simulink model "Copy_of_VTOLTiltrotor"  (R2024a)
settings: configuration reference "VTOLConfiguration" (kept outside this file)
undefined symbols (not defined in the file): airspeed, Battery, BCE12, BCE_Set_init, BMS_Controller_State, C, Cell10_P, Cell11_P, Cell12_P, Cell1_N, Cell1_P, Cell2_P, Cell3_P, Cell4_P, Cell5_P, Cell6_P, Cell7_P, Cell8_P, Cell9_P, Cell_Temperatures, Cell_Voltages, Charging_State, CityMission, control, controlParams, ControlSampleTime, CriticalTiltAngle, currentFactor, CV_Gain, ddx, ddy, ddz, Device_01, DiscIntNeverNeededParam, dx, dy, dz, Earth, env, F, F28379D_ADC_MaxCount, F28379D_ADC_Vmax, FixedWingMission, flightState, Foc_Ki_IxTcpu, Foc_Ki_S, Foc_Kp_I, Foc_Kp_S, fractalcoef, FSState, FWControlParams, HoverMission, I_cc, Ia_offset, Ib_offset, iniRoll, initPitch, iniYaw, IO334, IO334_DAC_Vmax ... (+55)
libraries: slrealtimeethercatlib x109, simulink x81, fl_lib x65, slpidlib x49, mcbcontrolslib x48, nesl_utility x43, speedgoatlib_hdlCoder_IO3xx x31, canmsglib x17, slrealtimeutilitieslib x13, mcbhdlplantlib x13, speedgoatlib_IO611 x12, dspstat3 x12
(part 18 of 20)

== system Copy_of_VTOLTiltrotor/Motor Control/Controller1/Controller_MIL/F28379D Firmware/Controller Algorithm/FOC/Speed Control MLD/PI_Controller_Speed ==
  Enable : Inport
  N_ref : Inport  Port=2
  N_fb : Inport  Port=3
  Kp_S : Inport  Port=4
  Ki_S : Inport  Port=5
  Discrete PI Controller with anti-windup & reset : slpidlib/PID Controller  Controller=PI  Form=Parallel  TimeDomain=Discrete-time  UseExternalTs=off  SampleTime=-1  IntegratorMethod=Forward Euler  FilterMethod=Forward Euler  ControllerParametersSource=external  P=1  I=1  UseKiTs=on  D=0  UseExternalDerivativeSource=off  N=100  UseFilter=on  TunerSelectOption=Transfer Function Based (PID Tuner App)  InitialConditionSource=external  InitialConditionForIntegrator=0  InitialConditionForFilter=0  DifferentiatorICPrevScaledInput=0  ExternalReset=level  TrackingMode=off  Kt=1  LimitOutput=on  SatLimitsSource=internal  UpperSaturationLimit=1  LowerSaturationLimit=-1  LinearizeAsGain=on  AntiWindupMode=clamping  Kb=1  LimitIntegrator=off  UpperIntegratorSaturationLimit=inf  LowerIntegratorSaturationLimit=-inf  RndMeth=Simplest  POutMin=[]  POutMax=[]  IOutMin=[]  IOutMax=[]  DOutMin=[]  DOutMax=[]  NOutMin=[]  NOutMax=[]  SumOutMin=[]  SumOutMax=[]  SaturationOutDataTypeStr=Inherit: Inherit via back propagation  SaturationOutMin=[]  SaturationOutMax=[]  PParamMin=[]  PParamMax=[]  IParamMin=[]  IParamMax=[]  DParamMin=[]  DParamMax=[]  NParamMin=[]  NParamMax=[]  KbParamMin=[]  KbParamMax=[]  KtParamMin=[]  KtParamMax=[]  KbOutMin=[]  KbOutMax=[]  KtOutMin=[]  KtOutMax=[]  IntegratorOutMin=[]  IntegratorOutMax=[]  FilterOutMin=[]  FilterOutMax=[]  SumI1OutMin=[]  SumI1OutMax=[]  SumI2OutMin=[]  SumI2OutMax=[]  SumI3OutMin=[]  SumI3OutMax=[]  SumI4OutMin=[]  SumI4OutMax=[]  SumDOutMin=[]  SumDOutMax=[]  DifferentiatorOutMin=[]  DifferentiatorOutMax=[]  FilterDiffOutCoefMin=[]  FilterDiffOutCoefMax=[]  ReciprocalOutMin=[]  ReciprocalOutMax=[]  SumDenOutMin=[]  SumDenOutMax=[]  SumNumOutMin=[]  SumNumOutMax=[]  DivideOutMin=[]  DivideOutMax=[]  UdiffTsProdOutMin=[]  UdiffTsProdOutMax=[]  NTsProdOutMin=[]  NTsProdOutMax=[]  UintegralTsProdOutMin=[]  UintegralTsProdOutMax=[]  UngainTsProdOutMin=[]  UngainTsProdOutMax=[]  ClampingZeroOutDataTypeStr=Inherit: Inherit via back propagation  ClampingZeroOutMin=[]  ClampingZeroOutMax=[]  FilterDenConstantOutDataTypeStr=Inherit: Inherit via back propagation  FilterDenConstantOutMin=[]  FilterDenConstantOutMax=[]  PCopyOutDataTypeStr=Inherit: Inherit via back propagation  PCopyOutMin=[]  PCopyOutMax=[]  NCopyOutDataTypeStr=Inherit: Inherit via back propagation  NCopyOutMin=[]  NCopyOutMax=[]  IntegratorContinuousStateAttributes=''  IntegratorStateMustResolveToSignalObject=off  IntegratorRTWStateStorageClass=Auto  FilterContinuousStateAttributes=''  FilterStateMustResolveToSignalObject=off  FilterRTWStateStorageClass=Auto  ParallelPVariant=ExternalParameters  IdealPVariant=Disabled  IVariant=ExternalParameters  DVariant=Disabled  IntegratorVariant=Discrete  SatVariant=Enabled  AWVariant=DiscClampingParallel  PCopyVariant=Disabled  TRVariant=Disabled  FdbkBlocksVariant=Forward  IdealPFdbkVariant=Disabled  SatFdbkVariant=Disabled  DerivativeFilterVariant=Disabled  NVariant=Disabled  NCopyVariant=Disabled_SignalSpec  FilterICVariant=Disabled  IntegratorICVariant=ExternalICs  ExternalResetVariant=ExternalReset  TRSumVariant=Passthrough  SumFdbkVariant=Disabled  SumVariant=Sum_PI  TsampFilterVariant=InternalTs  TsampNgainVariant=Passthrough  TsampIntegralVariant=Disabled_SignalSpec  ExternalSaturationOutDataTypeStr=Inherit: Same as second input  DerivativeSourceVariant=Disabled
  Ki2 : Constant  Value=0  OutDataTypeStr=single  SampleTime=-1
  Logical Operator : Logic  Operator=NOT  IconShape=distinctive  AllPortsSameDT=off  OutDataTypeStr=boolean
  Sum : Sum  Inputs=|+-  OutDataTypeStr=Inherit: Same as first input
  Iq_ref : Outport  VectorParamsAs1DForOutWhenUnconnected=off
  wires:
  Ki_S/1 -> Discrete PI Controller with anti-windup & reset/3
  Kp_S/1 -> Discrete PI Controller with anti-windup & reset/2
  Enable/1 -> Logical Operator/1
  Ki2/1 -> Discrete PI Controller with anti-windup & reset/5
  Logical Operator/1 -> Discrete PI Controller with anti-windup & reset/4
  Sum/1 -> Discrete PI Controller with anti-windup & reset/1
  N_ref/1 -> Sum/1
  N_fb/1 -> Sum/2
  Discrete PI Controller with anti-windup & reset/1 -> Iq_ref/1

== system Copy_of_VTOLTiltrotor/Motor Control/Controller1/Controller_MIL/F28379D Firmware/Controller Algorithm/FOC/Speed Control MLD/Speed_Ref_Selector ==
  Enable : Inport
  SpeedCommand : Inport  Port=2
  Speed_Ref_Open : Inport  Port=3
  IIR Filter : mcbcontrolslib/IIR Filter  VariantControl=Low Pass Filter  VariantSelect=Low-pass  FilterConstantInputType=Specify via dialog  Filter_constant=0.01  advancedSettings=off  Ts=50e-6  cutOff_freq=32.1525
  Switch : Switch  Criteria=u2 > Threshold  Threshold=0.5  SaturateOnIntegerOverflow=off  InputSameDT=off
  Speed_Ref_PU : Outport
  wires:
  SpeedCommand/1 -> Switch/1  "SpeedRef"
  Enable/1 -> Switch/2
  Speed_Ref_Open/1 -> Switch/3
  Switch/1 -> IIR Filter/1
  IIR Filter/1 -> Speed_Ref_PU/1

== system Copy_of_VTOLTiltrotor/Motor Control/Controller2/Controller_MIL/F28379D Firmware/Controller Algorithm/FOC/Current Control/Control_System ==
  Iab_meas_PU : Inport
  Pos_PU : Inport  Port=2
  Enable : Inport  Port=3
  Idq_ref_PU : Inport  Port=4
  SpeedRef : Inport  Port=5
  Kp_i : Inport  Port=6
  Ki_ixTcpu : Inport  Port=7
  Closed Loop Control : Subsystem
  Demux : Demux  Outputs=2
  NOT : Logic  Operator=NOT  IconShape=distinctive  AllPortsSameDT=off  OutDataTypeStr=boolean
  Open Loop Start-Up : Subsystem
  Output Scaling : Subsystem
  Switch : Switch  Criteria=u2 > Threshold  Threshold=0.5  SaturateOnIntegerOverflow=off  InputSameDT=off
  ModWave : Outport
  PWM_Enable : Outport  Port=2
  Idq_debug : Outport  Port=3  VectorParamsAs1DForOutWhenUnconnected=off
  wires:
  Open Loop Start-Up/1(PWM_Duty) -> Switch/3
  Switch/1 -> Output Scaling/1(PWM_Duty)
  Enable/1 -> Demux/1
  Demux/1 -> Closed Loop Control/Enable, Switch/2, NOT/1
  Demux/2 -> [EnablePWM], Open Loop Start-Up/1(<EnablePWM>)
  Iab_meas_PU/1 -> Closed Loop Control/1(Iab_meas_PU)
  Pos_PU/1 -> Closed Loop Control/2(Pos_PU)
  Idq_ref_PU/1 -> Closed Loop Control/3(Idq_ref_PU)  "idqref"
  [EnablePWM] -> Closed Loop Control/4(EnablePWM)
  Closed Loop Control/1(Idq_debug) -> Idq_debug/1
  Closed Loop Control/2(Vabc in PU) -> Switch/1
  Output Scaling/1(ModWave) -> ModWave/1
  Output Scaling/2(PWM_Enable) -> PWM_Enable/1
  [EnablePWM] -> Output Scaling/2(Enable)
  SpeedRef/1 -> Open Loop Start-Up/2(SpeedRef)
  NOT/1 -> Open Loop Start-Up/Enable
  Ki_ixTcpu/1 -> Closed Loop Control/6(Ki_ixTcpu)
  Kp_i/1 -> Closed Loop Control/5(Kp_i)

== system Copy_of_VTOLTiltrotor/Motor Control/Controller2/Controller_MIL/F28379D Firmware/Controller Algorithm/FOC/Speed Control MLD/PI_Controller_Speed ==
  Enable : Inport
  N_ref : Inport  Port=2
  N_fb : Inport  Port=3
  Kp_S : Inport  Port=4
  Ki_S : Inport  Port=5
  Discrete PI Controller with anti-windup & reset : slpidlib/PID Controller  Controller=PI  Form=Parallel  TimeDomain=Discrete-time  UseExternalTs=off  SampleTime=-1  IntegratorMethod=Forward Euler  FilterMethod=Forward Euler  ControllerParametersSource=external  P=1  I=1  UseKiTs=on  D=0  UseExternalDerivativeSource=off  N=100  UseFilter=on  TunerSelectOption=Transfer Function Based (PID Tuner App)  InitialConditionSource=external  InitialConditionForIntegrator=0  InitialConditionForFilter=0  DifferentiatorICPrevScaledInput=0  ExternalReset=level  TrackingMode=off  Kt=1  LimitOutput=on  SatLimitsSource=internal  UpperSaturationLimit=1  LowerSaturationLimit=-1  LinearizeAsGain=on  AntiWindupMode=clamping  Kb=1  LimitIntegrator=off  UpperIntegratorSaturationLimit=inf  LowerIntegratorSaturationLimit=-inf  RndMeth=Simplest  POutMin=[]  POutMax=[]  IOutMin=[]  IOutMax=[]  DOutMin=[]  DOutMax=[]  NOutMin=[]  NOutMax=[]  SumOutMin=[]  SumOutMax=[]  SaturationOutDataTypeStr=Inherit: Inherit via back propagation  SaturationOutMin=[]  SaturationOutMax=[]  PParamMin=[]  PParamMax=[]  IParamMin=[]  IParamMax=[]  DParamMin=[]  DParamMax=[]  NParamMin=[]  NParamMax=[]  KbParamMin=[]  KbParamMax=[]  KtParamMin=[]  KtParamMax=[]  KbOutMin=[]  KbOutMax=[]  KtOutMin=[]  KtOutMax=[]  IntegratorOutMin=[]  IntegratorOutMax=[]  FilterOutMin=[]  FilterOutMax=[]  SumI1OutMin=[]  SumI1OutMax=[]  SumI2OutMin=[]  SumI2OutMax=[]  SumI3OutMin=[]  SumI3OutMax=[]  SumI4OutMin=[]  SumI4OutMax=[]  SumDOutMin=[]  SumDOutMax=[]  DifferentiatorOutMin=[]  DifferentiatorOutMax=[]  FilterDiffOutCoefMin=[]  FilterDiffOutCoefMax=[]  ReciprocalOutMin=[]  ReciprocalOutMax=[]  SumDenOutMin=[]  SumDenOutMax=[]  SumNumOutMin=[]  SumNumOutMax=[]  DivideOutMin=[]  DivideOutMax=[]  UdiffTsProdOutMin=[]  UdiffTsProdOutMax=[]  NTsProdOutMin=[]  NTsProdOutMax=[]  UintegralTsProdOutMin=[]  UintegralTsProdOutMax=[]  UngainTsProdOutMin=[]  UngainTsProdOutMax=[]  ClampingZeroOutDataTypeStr=Inherit: Inherit via back propagation  ClampingZeroOutMin=[]  ClampingZeroOutMax=[]  FilterDenConstantOutDataTypeStr=Inherit: Inherit via back propagation  FilterDenConstantOutMin=[]  FilterDenConstantOutMax=[]  PCopyOutDataTypeStr=Inherit: Inherit via back propagation  PCopyOutMin=[]  PCopyOutMax=[]  NCopyOutDataTypeStr=Inherit: Inherit via back propagation  NCopyOutMin=[]  NCopyOutMax=[]  IntegratorContinuousStateAttributes=''  IntegratorStateMustResolveToSignalObject=off  IntegratorRTWStateStorageClass=Auto  FilterContinuousStateAttributes=''  FilterStateMustResolveToSignalObject=off  FilterRTWStateStorageClass=Auto  ParallelPVariant=ExternalParameters  IdealPVariant=Disabled  IVariant=ExternalParameters  DVariant=Disabled  IntegratorVariant=Discrete  SatVariant=Enabled  AWVariant=DiscClampingParallel  PCopyVariant=Disabled  TRVariant=Disabled  FdbkBlocksVariant=Forward  IdealPFdbkVariant=Disabled  SatFdbkVariant=Disabled  DerivativeFilterVariant=Disabled  NVariant=Disabled  NCopyVariant=Disabled_SignalSpec  FilterICVariant=Disabled  IntegratorICVariant=ExternalICs  ExternalResetVariant=ExternalReset  TRSumVariant=Passthrough  SumFdbkVariant=Disabled  SumVariant=Sum_PI  TsampFilterVariant=InternalTs  TsampNgainVariant=Passthrough  TsampIntegralVariant=Disabled_SignalSpec  ExternalSaturationOutDataTypeStr=Inherit: Same as second input  DerivativeSourceVariant=Disabled
  Ki2 : Constant  Value=0  OutDataTypeStr=single  SampleTime=-1
  Logical Operator : Logic  Operator=NOT  IconShape=distinctive  AllPortsSameDT=off  OutDataTypeStr=boolean
  Sum : Sum  Inputs=|+-  OutDataTypeStr=Inherit: Same as first input
  Iq_ref : Outport  VectorParamsAs1DForOutWhenUnconnected=off
  wires:
  Ki_S/1 -> Discrete PI Controller with anti-windup & reset/3
  Kp_S/1 -> Discrete PI Controller with anti-windup & reset/2
  Enable/1 -> Logical Operator/1
  Ki2/1 -> Discrete PI Controller with anti-windup & reset/5
  Logical Operator/1 -> Discrete PI Controller with anti-windup & reset/4
  Sum/1 -> Discrete PI Controller with anti-windup & reset/1
  N_ref/1 -> Sum/1
  N_fb/1 -> Sum/2
  Discrete PI Controller with anti-windup & reset/1 -> Iq_ref/1

== system Copy_of_VTOLTiltrotor/Motor Control/Controller2/Controller_MIL/F28379D Firmware/Controller Algorithm/FOC/Speed Control MLD/Speed_Ref_Selector ==
  Enable : Inport
  SpeedCommand : Inport  Port=2
  Speed_Ref_Open : Inport  Port=3
  IIR Filter : mcbcontrolslib/IIR Filter  VariantControl=Low Pass Filter  VariantSelect=Low-pass  FilterConstantInputType=Specify via dialog  Filter_constant=0.01  advancedSettings=off  Ts=50e-6  cutOff_freq=32.1525
  Switch : Switch  Criteria=u2 > Threshold  Threshold=0.5  SaturateOnIntegerOverflow=off  InputSameDT=off
  Speed_Ref_PU : Outport
  wires:
  SpeedCommand/1 -> Switch/1  "SpeedRef"
  Enable/1 -> Switch/2
  Speed_Ref_Open/1 -> Switch/3
  Switch/1 -> IIR Filter/1
  IIR Filter/1 -> Speed_Ref_PU/1

== system Copy_of_VTOLTiltrotor/Motor Control/Controller3/Controller_MIL/F28379D Firmware/Controller Algorithm/FOC/Current Control/Control_System ==
  Iab_meas_PU : Inport
  Pos_PU : Inport  Port=2
  Enable : Inport  Port=3
  Idq_ref_PU : Inport  Port=4
  SpeedRef : Inport  Port=5
  Kp_i : Inport  Port=6
  Ki_ixTcpu : Inport  Port=7
  Closed Loop Control : Subsystem
  Demux : Demux  Outputs=2
  NOT : Logic  Operator=NOT  IconShape=distinctive  AllPortsSameDT=off  OutDataTypeStr=boolean
  Open Loop Start-Up : Subsystem
  Output Scaling : Subsystem
  Switch : Switch  Criteria=u2 > Threshold  Threshold=0.5  SaturateOnIntegerOverflow=off  InputSameDT=off
  ModWave : Outport
  PWM_Enable : Outport  Port=2
  Idq_debug : Outport  Port=3  VectorParamsAs1DForOutWhenUnconnected=off
  wires:
  Open Loop Start-Up/1(PWM_Duty) -> Switch/3
  Switch/1 -> Output Scaling/1(PWM_Duty)
  Enable/1 -> Demux/1
  Demux/1 -> Closed Loop Control/Enable, Switch/2, NOT/1
  Demux/2 -> [EnablePWM], Open Loop Start-Up/1(<EnablePWM>)
  Iab_meas_PU/1 -> Closed Loop Control/1(Iab_meas_PU)
  Pos_PU/1 -> Closed Loop Control/2(Pos_PU)
  Idq_ref_PU/1 -> Closed Loop Control/3(Idq_ref_PU)  "idqref"
  [EnablePWM] -> Closed Loop Control/4(EnablePWM)
  Closed Loop Control/1(Idq_debug) -> Idq_debug/1
  Closed Loop Control/2(Vabc in PU) -> Switch/1
  Output Scaling/1(ModWave) -> ModWave/1
  Output Scaling/2(PWM_Enable) -> PWM_Enable/1
  [EnablePWM] -> Output Scaling/2(Enable)
  SpeedRef/1 -> Open Loop Start-Up/2(SpeedRef)
  NOT/1 -> Open Loop Start-Up/Enable
  Ki_ixTcpu/1 -> Closed Loop Control/6(Ki_ixTcpu)
  Kp_i/1 -> Closed Loop Control/5(Kp_i)

== system Copy_of_VTOLTiltrotor/Motor Control/Controller3/Controller_MIL/F28379D Firmware/Controller Algorithm/FOC/Speed Control MLD/PI_Controller_Speed ==
  Enable : Inport
  N_ref : Inport  Port=2
  N_fb : Inport  Port=3
  Kp_S : Inport  Port=4
  Ki_S : Inport  Port=5
  Discrete PI Controller with anti-windup & reset : slpidlib/PID Controller  Controller=PI  Form=Parallel  TimeDomain=Discrete-time  UseExternalTs=off  SampleTime=-1  IntegratorMethod=Forward Euler  FilterMethod=Forward Euler  ControllerParametersSource=external  P=1  I=1  UseKiTs=on  D=0  UseExternalDerivativeSource=off  N=100  UseFilter=on  TunerSelectOption=Transfer Function Based (PID Tuner App)  InitialConditionSource=external  InitialConditionForIntegrator=0  InitialConditionForFilter=0  DifferentiatorICPrevScaledInput=0  ExternalReset=level  TrackingMode=off  Kt=1  LimitOutput=on  SatLimitsSource=internal  UpperSaturationLimit=1  LowerSaturationLimit=-1  LinearizeAsGain=on  AntiWindupMode=clamping  Kb=1  LimitIntegrator=off  UpperIntegratorSaturationLimit=inf  LowerIntegratorSaturationLimit=-inf  RndMeth=Simplest  POutMin=[]  POutMax=[]  IOutMin=[]  IOutMax=[]  DOutMin=[]  DOutMax=[]  NOutMin=[]  NOutMax=[]  SumOutMin=[]  SumOutMax=[]  SaturationOutDataTypeStr=Inherit: Inherit via back propagation  SaturationOutMin=[]  SaturationOutMax=[]  PParamMin=[]  PParamMax=[]  IParamMin=[]  IParamMax=[]  DParamMin=[]  DParamMax=[]  NParamMin=[]  NParamMax=[]  KbParamMin=[]  KbParamMax=[]  KtParamMin=[]  KtParamMax=[]  KbOutMin=[]  KbOutMax=[]  KtOutMin=[]  KtOutMax=[]  IntegratorOutMin=[]  IntegratorOutMax=[]  FilterOutMin=[]  FilterOutMax=[]  SumI1OutMin=[]  SumI1OutMax=[]  SumI2OutMin=[]  SumI2OutMax=[]  SumI3OutMin=[]  SumI3OutMax=[]  SumI4OutMin=[]  SumI4OutMax=[]  SumDOutMin=[]  SumDOutMax=[]  DifferentiatorOutMin=[]  DifferentiatorOutMax=[]  FilterDiffOutCoefMin=[]  FilterDiffOutCoefMax=[]  ReciprocalOutMin=[]  ReciprocalOutMax=[]  SumDenOutMin=[]  SumDenOutMax=[]  SumNumOutMin=[]  SumNumOutMax=[]  DivideOutMin=[]  DivideOutMax=[]  UdiffTsProdOutMin=[]  UdiffTsProdOutMax=[]  NTsProdOutMin=[]  NTsProdOutMax=[]  UintegralTsProdOutMin=[]  UintegralTsProdOutMax=[]  UngainTsProdOutMin=[]  UngainTsProdOutMax=[]  ClampingZeroOutDataTypeStr=Inherit: Inherit via back propagation  ClampingZeroOutMin=[]  ClampingZeroOutMax=[]  FilterDenConstantOutDataTypeStr=Inherit: Inherit via back propagation  FilterDenConstantOutMin=[]  FilterDenConstantOutMax=[]  PCopyOutDataTypeStr=Inherit: Inherit via back propagation  PCopyOutMin=[]  PCopyOutMax=[]  NCopyOutDataTypeStr=Inherit: Inherit via back propagation  NCopyOutMin=[]  NCopyOutMax=[]  IntegratorContinuousStateAttributes=''  IntegratorStateMustResolveToSignalObject=off  IntegratorRTWStateStorageClass=Auto  FilterContinuousStateAttributes=''  FilterStateMustResolveToSignalObject=off  FilterRTWStateStorageClass=Auto  ParallelPVariant=ExternalParameters  IdealPVariant=Disabled  IVariant=ExternalParameters  DVariant=Disabled  IntegratorVariant=Discrete  SatVariant=Enabled  AWVariant=DiscClampingParallel  PCopyVariant=Disabled  TRVariant=Disabled  FdbkBlocksVariant=Forward  IdealPFdbkVariant=Disabled  SatFdbkVariant=Disabled  DerivativeFilterVariant=Disabled  NVariant=Disabled  NCopyVariant=Disabled_SignalSpec  FilterICVariant=Disabled  IntegratorICVariant=ExternalICs  ExternalResetVariant=ExternalReset  TRSumVariant=Passthrough  SumFdbkVariant=Disabled  SumVariant=Sum_PI  TsampFilterVariant=InternalTs  TsampNgainVariant=Passthrough  TsampIntegralVariant=Disabled_SignalSpec  ExternalSaturationOutDataTypeStr=Inherit: Same as second input  DerivativeSourceVariant=Disabled
  Ki2 : Constant  Value=0  OutDataTypeStr=single  SampleTime=-1
  Logical Operator : Logic  Operator=NOT  IconShape=distinctive  AllPortsSameDT=off  OutDataTypeStr=boolean
  Sum : Sum  Inputs=|+-  OutDataTypeStr=Inherit: Same as first input
  Iq_ref : Outport  VectorParamsAs1DForOutWhenUnconnected=off
  wires:
  Ki_S/1 -> Discrete PI Controller with anti-windup & reset/3
  Kp_S/1 -> Discrete PI Controller with anti-windup & reset/2
  Enable/1 -> Logical Operator/1
  Ki2/1 -> Discrete PI Controller with anti-windup & reset/5
  Logical Operator/1 -> Discrete PI Controller with anti-windup & reset/4
  Sum/1 -> Discrete PI Controller with anti-windup & reset/1
  N_ref/1 -> Sum/1
  N_fb/1 -> Sum/2
  Discrete PI Controller with anti-windup & reset/1 -> Iq_ref/1

== system Copy_of_VTOLTiltrotor/Motor Control/Controller3/Controller_MIL/F28379D Firmware/Controller Algorithm/FOC/Speed Control MLD/Speed_Ref_Selector ==
  Enable : Inport
  SpeedCommand : Inport  Port=2
  Speed_Ref_Open : Inport  Port=3
  IIR Filter : mcbcontrolslib/IIR Filter  VariantControl=Low Pass Filter  VariantSelect=Low-pass  FilterConstantInputType=Specify via dialog  Filter_constant=0.01  advancedSettings=off  Ts=50e-6  cutOff_freq=32.1525
  Switch : Switch  Criteria=u2 > Threshold  Threshold=0.5  SaturateOnIntegerOverflow=off  InputSameDT=off
  Speed_Ref_PU : Outport
  wires:
  SpeedCommand/1 -> Switch/1  "SpeedRef"
  Enable/1 -> Switch/2
  Speed_Ref_Open/1 -> Switch/3
  Switch/1 -> IIR Filter/1
  IIR Filter/1 -> Speed_Ref_PU/1

== system Copy_of_VTOLTiltrotor/Battery Management System/Battery/HW Interface/BCE - HIL/Battery Cell Emulator/BCE Write /Subsystem/BCE Write /Enable until confirmed ==
  global enable : Inport
  D1 : Inport  Port=2
  D2 : Inport  Port=3
  D3 : Inport  Port=4
  D4 : Inport  Port=5
  D5 : Inport  Port=6
  D6 : Inport  Port=7
  D7 : Inport  Port=8
  D8 : Inport  Port=9
  D9 : Inport  Port=10
  D10 : Inport  Port=11
  D11 : Inport  Port=12
  D12 : Inport  Port=13
  Compare To Constant{,1..11} (12 alike) : simulink/Logic and Bit Operations/Compare To Constant  relop===  const=2  OutDataTypeStr=boolean
  Data Type Conversion : DataTypeConversion  OutDataTypeStr=int32  SaturateOnIntegerOverflow=off  RndMeth=Floor
  Logical Operator : Logic  Operator=NAND  Inputs=12  AllPortsSameDT=off  OutDataTypeStr=boolean
  Logical Operator1 : Logic  AllPortsSameDT=off  OutDataTypeStr=boolean
  Logical Operator2 : Logic  Operator=NOT  AllPortsSameDT=off  OutDataTypeStr=boolean
  MinMax Running Resettable{,1..11} (12 alike) : simulink/Math Operations/MinMax Running Resettable  Function=max  vinit=0.0
  Unit Delay : UnitDelay  SampleTime=-1  HasFrameUpgradeWarning=on
  Out1 : Outport
  wires:
  Logical Operator2/1 -> MinMax Running Resettable/2, MinMax Running Resettable1/2, MinMax Running Resettable2/2, MinMax Running Resettable3/2, MinMax Running Resettable4/2, MinMax Running Resettable5/2, MinMax Running Resettable6/2, MinMax Running Resettable7/2, MinMax Running Resettable8/2, MinMax Running Resettable9/2, MinMax Running Resettable10/2, MinMax Running Resettable11/2
  D12/1 -> Compare To Constant11/1
  D6/1 -> Compare To Constant5/1
  D1/1 -> Compare To Constant/1
  D5/1 -> Compare To Constant4/1
  MinMax Running Resettable11/1 -> Logical Operator/12
  MinMax Running Resettable10/1 -> Logical Operator/11
  Compare To Constant4/1 -> MinMax Running Resettable4/1
  MinMax Running Resettable1/1 -> Logical Operator/2
  MinMax Running Resettable8/1 -> Logical Operator/9
  MinMax Running Resettable3/1 -> Logical Operator/4
  Compare To Constant7/1 -> MinMax Running Resettable7/1
  MinMax Running Resettable2/1 -> Logical Operator/3
  Compare To Constant2/1 -> MinMax Running Resettable2/1
  D10/1 -> Compare To Constant9/1
  Compare To Constant3/1 -> MinMax Running Resettable3/1
  D8/1 -> Compare To Constant7/1
  MinMax Running Resettable9/1 -> Logical Operator/10
  MinMax Running Resettable7/1 -> Logical Operator/8
  MinMax Running Resettable6/1 -> Logical Operator/7
  Compare To Constant1/1 -> MinMax Running Resettable1/1
  MinMax Running Resettable5/1 -> Logical Operator/6
  D2/1 -> Compare To Constant1/1
  D7/1 -> Compare To Constant6/1
  Compare To Constant/1 -> MinMax Running Resettable/1
  MinMax Running Resettable4/1 -> Logical Operator/5
  D3/1 -> Compare To Constant2/1
  Compare To Constant9/1 -> MinMax Running Resettable9/1
  Compare To Constant5/1 -> MinMax Running Resettable5/1
  Compare To Constant10/1 -> MinMax Running Resettable10/1
  Data Type Conversion/1 -> Out1/1
  Compare To Constant8/1 -> MinMax Running Resettable8/1
  MinMax Running Resettable/1 -> Logical Operator/1
  D9/1 -> Compare To Constant8/1
  D4/1 -> Compare To Constant3/1
  Compare To Constant6/1 -> MinMax Running Resettable6/1
  D11/1 -> Compare To Constant10/1
  Compare To Constant11/1 -> MinMax Running Resettable11/1
  Logical Operator1/1 -> Data Type Conversion/1
  Unit Delay/1 -> Logical Operator1/2
  Logical Operator/1 -> Unit Delay/1
  global enable/1 -> Logical Operator2/1, Logical Operator1/1

== system Copy_of_VTOLTiltrotor/Dynamics/Force and Moments/Aerodynamic Forces/Compute Body Frame Forces and Moments/Wind frame F& M/Lateral Channel/CY/roll factors/Subsystem ==
  r : Inport
  Airspeed : Inport  Port=2
  Cmq3 : Constant
      settings: AttributesFormatString=%<Value>
  Cmq4 : Constant  Value=uavParam.geom.b
      settings: AttributesFormatString=%<Value>
  Gain : Gain  Gain=2
  Product1 : Product  Inputs=***/  SaturateOnIntegerOverflow=on  OutDataTypeStr=Inherit: Same as first input
  Saturation : Saturate  UpperLimit=inf  LowerLimit=0.1
      settings: AttributesFormatString="[%<LowerLimit>  %<UpperLimit>]"
  Yaw Rate Fac : Outport  VectorParamsAs1DForOutWhenUnconnected=off
  wires:
  Saturation/1 -> Gain/1
  Cmq4/1 -> Product1/3
  Airspeed/1 -> Saturation/1
  Gain/1 -> Product1/4
  Cmq3/1 -> Product1/2
  Product1/1 -> Yaw Rate Fac/1
  r/1 -> Product1/1

== system Copy_of_VTOLTiltrotor/Dynamics/Force and Moments/Aerodynamic Forces/Compute Body Frame Forces and Moments/Wind frame F& M/Lateral Channel/CY/roll factors/roll rate fact ==
  p : Inport
  Airspeed : Inport  Port=2
  Cmq1 : Constant
      settings: AttributesFormatString=%<Value>
  Cmq2 : Constant  Value=uavParam.geom.b
      settings: AttributesFormatString=%<Value>
  Gain : Gain  Gain=2
  Product : Product  Inputs=***/  SaturateOnIntegerOverflow=on  OutDataTypeStr=Inherit: Same as first input
  Saturation : Saturate  UpperLimit=inf  LowerLimit=0.1
      settings: AttributesFormatString="[%<LowerLimit>  %<UpperLimit>]"
  Roll Rate Fac : Outport  VectorParamsAs1DForOutWhenUnconnected=off
  wires:
  Airspeed/1 -> Saturation/1
  Cmq2/1 -> Product/3
  Cmq1/1 -> Product/2
  p/1 -> Product/1
  Product/1 -> Roll Rate Fac/1
  Saturation/1 -> Gain/1
  Gain/1 -> Product/4

== system Copy_of_VTOLTiltrotor/Dynamics/Force and Moments/Aerodynamic Forces/Compute Body Frame Forces and Moments/Wind frame F& M/Lateral Channel/Cl/roll factors/roll rate fact ==
  p : Inport
  Airspeed : Inport  Port=2
  Cmq1 : Constant  Value=.5
      settings: AttributesFormatString=%<Value>
  Cmq2 : Constant  Value=uavParam.geom.b
      settings: AttributesFormatString=%<Value>
  Product : Product  Inputs=***/  SaturateOnIntegerOverflow=on  OutDataTypeStr=Inherit: Same as first input
  Saturation : Saturate  UpperLimit=inf  LowerLimit=0.1
      settings: AttributesFormatString="[%<LowerLimit>  %<UpperLimit>]"
  Roll Rate Fac : Outport  VectorParamsAs1DForOutWhenUnconnected=off
  wires:
  Saturation/1 -> Product/4
  Airspeed/1 -> Saturation/1
  Cmq2/1 -> Product/3
  Cmq1/1 -> Product/2
  p/1 -> Product/1
  Product/1 -> Roll Rate Fac/1

== system Copy_of_VTOLTiltrotor/Dynamics/Force and Moments/Aerodynamic Forces/Compute Body Frame Forces and Moments/Wind frame F& M/Lateral Channel/Cn/yaw factors/roll rate fact ==
  p : Inport
  Airspeed : Inport  Port=2
  Cmq1 : Constant  Value=.5
      settings: AttributesFormatString=%<Value>
  Cmq2 : Constant  Value=uavParam.geom.b
      settings: AttributesFormatString=%<Value>
  Product : Product  Inputs=***/  SaturateOnIntegerOverflow=on  OutDataTypeStr=Inherit: Same as first input
  Saturation : Saturate  UpperLimit=inf  LowerLimit=0.1
      settings: AttributesFormatString="[%<LowerLimit>  %<UpperLimit>]"
  Roll Rate Fac : Outport  VectorParamsAs1DForOutWhenUnconnected=off
  wires:
  Saturation/1 -> Product/4
  Airspeed/1 -> Saturation/1
  Cmq2/1 -> Product/3
  Cmq1/1 -> Product/2
  p/1 -> Product/1
  Product/1 -> Roll Rate Fac/1

== system Copy_of_VTOLTiltrotor/Dynamics/Force and Moments/Aerodynamic Forces/Compute Body Frame Forces and Moments/Wind frame F& M/Longitudinal Channel/CL/Lift due to pitch rate/pitch rate factor ==
  q : Inport
  Airspeed : Inport  Port=2
  Cmq2 : Constant  Value=uavParam.geom.c
      settings: AttributesFormatString=%<Value>
  Gain : Gain  Gain=2
  Product : Product  Inputs=**/  SaturateOnIntegerOverflow=on  OutDataTypeStr=Inherit: Same as first input
  Saturation : Saturate  UpperLimit=inf  LowerLimit=0.1
      settings: AttributesFormatString="[%<LowerLimit>  %<UpperLimit>]"
  Pitch Rate Fac : Outport  VectorParamsAs1DForOutWhenUnconnected=off
  wires:
  Cmq2/1 -> Product/2
  Airspeed/1 -> Saturation/1
  q/1 -> Product/1
  Product/1 -> Pitch Rate Fac/1
  Saturation/1 -> Gain/1
  Gain/1 -> Product/3

== system Copy_of_VTOLTiltrotor/Dynamics/Force and Moments/Aerodynamic Forces/Compute Body Frame Forces and Moments/Wind frame F& M/Longitudinal Channel/Cm/Lift due to pitch rate/pitch rate factor ==
  q : Inport
  Airspeed : Inport  Port=2
  Cmq2 : Constant  Value=uavParam.geom.c
      settings: AttributesFormatString=%<Value>
  Gain : Gain  Gain=2
  Product : Product  Inputs=**/  SaturateOnIntegerOverflow=on  OutDataTypeStr=Inherit: Same as first input
  Saturation : Saturate  UpperLimit=inf  LowerLimit=0.1
      settings: AttributesFormatString="[%<LowerLimit>  %<UpperLimit>]"
  Pitch Rate Fac : Outport  VectorParamsAs1DForOutWhenUnconnected=off
  wires:
  Cmq2/1 -> Product/2
  Airspeed/1 -> Saturation/1
  q/1 -> Product/1
  Product/1 -> Pitch Rate Fac/1
  Saturation/1 -> Gain/1
  Gain/1 -> Product/3

== system Copy_of_VTOLTiltrotor/Flight Controller/Guidance Test Bench/ControlType/Guidance Testbench/Guidance Logic/Guidance Stateflow/Guidance Mode Selector/GuidanceLogic.WP/Back Transition Guard/Triggered Subsystem ==
  Poses : Inport
  Trigger : TriggerPort  VariantControl=(inherit)
  Reshape : Reshape  OutputDimensionality=Customize  OutputDimensions=[3,1]
  Selector : Selector  InputPortWidth=4  IndexOptions=Index vector (dialog)  Indices=[1 2 3]  OutputSizes=1
  HoldPositionValue : Outport
  wires:
  Poses/1 -> Selector/1
  Selector/1 -> Reshape/1
  Reshape/1 -> HoldPositionValue/1

== system Copy_of_VTOLTiltrotor/Flight Controller/Guidance Test Bench/ControlType/Guidance Testbench/Guidance Logic/Guidance Stateflow/Guidance Mode Selector/GuidanceLogic.WP/Dist2WP/Subsystem ==
  V : Inport
  Dot Product1 : DotProduct  OutDataTypeStr=Inherit: Inherit via internal rule
  Product : Product  Inputs=*/
  Saturation : Saturate  UpperLimit=inf  LowerLimit=0.00001
  Sqrt : Sqrt
  V_unit : Outport
  wires:
  V/1 -> Dot Product1/2, Dot Product1/1, Product/1
  Sqrt/1 -> Product/2
  Dot Product1/1 -> Saturation/1
  Saturation/1 -> Sqrt/1
  Product/1 -> V_unit/1

== system Copy_of_VTOLTiltrotor/Motor Control/Controller/Controller_MIL/F28379D Firmware/Controller Algorithm/FOC/Current Control/Control_System/Closed Loop Control ==
  Iab_meas_PU : Inport
  Pos_PU : Inport  Port=2
  Idq_ref_PU : Inport  Port=3
  EnablePWM : Inport  Port=4
  Kp_i : Inport  Port=5
  Ki_ixTcpu : Inport  Port=6
  Enable : EnablePort
  Subsystem : Subsystem
  Terminator : Terminator
  Idq_debug : Outport
  Vabc in PU : Outport  Port=2
  wires:
  Subsystem/3(VI_fb) -> Terminator/1
  Idq_ref_PU/1 -> Subsystem/3(Idq_ref_PU)
  Iab_meas_PU/1 -> Subsystem/1(Iab_meas_PU)
  EnablePWM/1 -> Subsystem/4(EnablePWM)
  Pos_PU/1 -> Subsystem/2(Pos_PU)
  Subsystem/2(VIdq_debug) -> Idq_debug/1
  Subsystem/1(Vabc in PU) -> Vabc in PU/1
  Ki_ixTcpu/1 -> Subsystem/6(Ki_ixTcpu)
  Kp_i/1 -> Subsystem/5(Kp_i)

== system Copy_of_VTOLTiltrotor/Motor Control/Controller/Controller_MIL/F28379D Firmware/Controller Algorithm/FOC/Current Control/Control_System/Open Loop Start-Up ==
  <EnablePWM> : Inport
  SpeedRef : Inport  Port=2
  Enable : EnablePort
  3-Phase Sine Voltage Generator : mcbcontrolslib/3-Phase Sine Voltage Generator  AngleInput=Radians  N_points=1024
  Abs : Abs  SaturateOnIntegerOverflow=off
  Correction_Factor_sinePWM : Gain  Gain=2/sqrt(3)  RndMeth=Simplest  OutDataTypeStr=Inherit: Same as input
  Gain : Gain  Gain=1000
  Mux1 : Mux  Inputs=3
  PU2freq : Gain  Gain=PU_System_N_base *Maxon_645604_Np/60  RndMeth=Simplest  OutDataTypeStr=Inherit: Same as input
  Position Generator : mcbcontrolslib/Position Generator  AngleOutput=Radians  ExternalReset=none  Offset=0
  Product : Product  RndMeth=Simplest  OutDataTypeStr=Inherit: Same as first input
  Ramp Generator : Subsystem
  Ramp_Time (sec) : Constant  Value=0.0025  OutDataTypeStr=single  SampleTime=-1
  Rate Limiter : mcbcontrolslib/IIR Filter  VariantControl=Low Pass Filter  VariantSelect=Low-pass  FilterConstantInputType=Specify via dialog  Filter_constant=0.0001  advancedSettings=off  Ts=50e-6  cutOff_freq=0.31834
  Saturation : Saturate  UpperLimit=0.95  LowerLimit=0.15  RndMeth=Simplest
  V-by-f : Gain  Gain=1/(PU_System_N_base*Maxon_645604_Np*2)  RndMeth=Simplest  OutDataTypeStr=Inherit: Same as input
  position_increment : Gain  Gain=2*pi*Ts_CPU  RndMeth=Simplest  OutDataTypeStr=Inherit: Same as input
  PWM_Duty : Outport  VectorParamsAs1DForOutWhenUnconnected=off
  wires:
  3-Phase Sine Voltage Generator/1 -> Mux1/1
  3-Phase Sine Voltage Generator/3 -> Mux1/3
  Position Generator/1 -> 3-Phase Sine Voltage Generator/2  "Eps"
  Saturation/1 -> 3-Phase Sine Voltage Generator/1  "Amplitude"
  Mux1/1 -> PWM_Duty/1
  Ramp Generator/1(Ramp) -> Product/2
  Ramp_Time (sec)/1 -> Ramp Generator/1(Ramp_Time)
  Abs/1 -> V-by-f/1  "Frequency"
  position_increment/1 -> Position Generator/1
  V-by-f/1 -> Gain/1
  PU2freq/1 -> Rate Limiter/1
  Correction_Factor_sinePWM/1 -> Saturation/1
  3-Phase Sine Voltage Generator/2 -> Mux1/2
  <EnablePWM>/1 -> Ramp Generator/2(Enable)
  Product/1 -> Abs/1, position_increment/1
  Rate Limiter/1 -> Product/1
  SpeedRef/1 -> PU2freq/1
  Gain/1 -> Correction_Factor_sinePWM/1

== system Copy_of_VTOLTiltrotor/Motor Control/Controller/Controller_MIL/F28379D Firmware/Controller Algorithm/FOC/Current Control/Control_System/Output Scaling ==
  PWM_Duty : Inport
  Enable : Inport  Port=2
  Constant : Constant  Value=0.5  OutDataTypeStr=single
  Data Type Conversion : DataTypeConversion  OutDataTypeStr=single  SaturateOnIntegerOverflow=off  RndMeth=Floor
  Gain : Gain  Gain=0.5  OutDataTypeStr=Inherit: Same as input
  Sum : Sum  Inputs=|++
  ModWave : Outport
  PWM_Enable : Outport  Port=2
  wires:
  Sum/1 -> ModWave/1  "duty"
  Constant/1 -> Sum/2
  Gain/1 -> Sum/1  "ModWave"
  PWM_Duty/1 -> Gain/1
  Data Type Conversion/1 -> PWM_Enable/1
  Enable/1 -> Data Type Conversion/1

== system Copy_of_VTOLTiltrotor/Motor Control/Controller1/Controller_MIL/F28379D Firmware/Controller Algorithm/FOC/Current Control/Control_System/Closed Loop Control ==
  Iab_meas_PU : Inport
  Pos_PU : Inport  Port=2
  Idq_ref_PU : Inport  Port=3
  EnablePWM : Inport  Port=4
  Kp_i : Inport  Port=5
  Ki_ixTcpu : Inport  Port=6
  Enable : EnablePort
  Subsystem : Subsystem
  Terminator : Terminator
  Idq_debug : Outport
  Vabc in PU : Outport  Port=2
  wires:
  Subsystem/3(VI_fb) -> Terminator/1
  Idq_ref_PU/1 -> Subsystem/3(Idq_ref_PU)
  Iab_meas_PU/1 -> Subsystem/1(Iab_meas_PU)
  EnablePWM/1 -> Subsystem/4(EnablePWM)
  Pos_PU/1 -> Subsystem/2(Pos_PU)
  Subsystem/2(VIdq_debug) -> Idq_debug/1
  Subsystem/1(Vabc in PU) -> Vabc in PU/1
  Ki_ixTcpu/1 -> Subsystem/6(Ki_ixTcpu)
  Kp_i/1 -> Subsystem/5(Kp_i)

== system Copy_of_VTOLTiltrotor/Motor Control/Controller1/Controller_MIL/F28379D Firmware/Controller Algorithm/FOC/Current Control/Control_System/Open Loop Start-Up ==
  <EnablePWM> : Inport
  SpeedRef : Inport  Port=2
  Enable : EnablePort
  3-Phase Sine Voltage Generator : mcbcontrolslib/3-Phase Sine Voltage Generator  AngleInput=Radians  N_points=1024
  Abs : Abs  SaturateOnIntegerOverflow=off
  Correction_Factor_sinePWM : Gain  Gain=2/sqrt(3)  RndMeth=Simplest  OutDataTypeStr=Inherit: Same as input
  Gain : Gain  Gain=1000
  Mux1 : Mux  Inputs=3
  PU2freq : Gain  Gain=PU_System_N_base *Maxon_645604_Np/60  RndMeth=Simplest  OutDataTypeStr=Inherit: Same as input
  Position Generator : mcbcontrolslib/Position Generator  AngleOutput=Radians  ExternalReset=none  Offset=0
  Product : Product  RndMeth=Simplest  OutDataTypeStr=Inherit: Same as first input
  Ramp Generator : Subsystem
  Ramp_Time (sec) : Constant  Value=0.0025  OutDataTypeStr=single  SampleTime=-1
  Rate Limiter : mcbcontrolslib/IIR Filter  VariantControl=Low Pass Filter  VariantSelect=Low-pass  FilterConstantInputType=Specify via dialog  Filter_constant=0.0001  advancedSettings=off  Ts=50e-6  cutOff_freq=0.31834
  Saturation : Saturate  UpperLimit=0.95  LowerLimit=0.15  RndMeth=Simplest
  V-by-f : Gain  Gain=1/(PU_System_N_base*Maxon_645604_Np*2)  RndMeth=Simplest  OutDataTypeStr=Inherit: Same as input
  position_increment : Gain  Gain=2*pi*Ts_CPU  RndMeth=Simplest  OutDataTypeStr=Inherit: Same as input
  PWM_Duty : Outport  VectorParamsAs1DForOutWhenUnconnected=off
  wires:
  3-Phase Sine Voltage Generator/1 -> Mux1/1
  3-Phase Sine Voltage Generator/3 -> Mux1/3
  Position Generator/1 -> 3-Phase Sine Voltage Generator/2  "Eps"
  Saturation/1 -> 3-Phase Sine Voltage Generator/1  "Amplitude"
  Mux1/1 -> PWM_Duty/1
  Ramp Generator/1(Ramp) -> Product/2
  Ramp_Time (sec)/1 -> Ramp Generator/1(Ramp_Time)
  Abs/1 -> V-by-f/1  "Frequency"
  position_increment/1 -> Position Generator/1
  V-by-f/1 -> Gain/1
  PU2freq/1 -> Rate Limiter/1
  Correction_Factor_sinePWM/1 -> Saturation/1
  3-Phase Sine Voltage Generator/2 -> Mux1/2
  <EnablePWM>/1 -> Ramp Generator/2(Enable)
  Product/1 -> Abs/1, position_increment/1
  Rate Limiter/1 -> Product/1
  SpeedRef/1 -> PU2freq/1
  Gain/1 -> Correction_Factor_sinePWM/1

== system Copy_of_VTOLTiltrotor/Motor Control/Controller1/Controller_MIL/F28379D Firmware/Controller Algorithm/FOC/Current Control/Control_System/Output Scaling ==
  PWM_Duty : Inport
  Enable : Inport  Port=2
  Constant : Constant  Value=0.5  OutDataTypeStr=single
  Data Type Conversion : DataTypeConversion  OutDataTypeStr=single  SaturateOnIntegerOverflow=off  RndMeth=Floor
  Gain : Gain  Gain=0.5  OutDataTypeStr=Inherit: Same as input
  Sum : Sum  Inputs=|++
  ModWave : Outport
  PWM_Enable : Outport  Port=2
  wires:
  Sum/1 -> ModWave/1  "duty"
  Constant/1 -> Sum/2
  Gain/1 -> Sum/1  "ModWave"
  PWM_Duty/1 -> Gain/1
  Data Type Conversion/1 -> PWM_Enable/1
  Enable/1 -> Data Type Conversion/1

== system Copy_of_VTOLTiltrotor/Motor Control/Controller2/Controller_MIL/F28379D Firmware/Controller Algorithm/FOC/Current Control/Control_System/Closed Loop Control ==
  Iab_meas_PU : Inport
  Pos_PU : Inport  Port=2
  Idq_ref_PU : Inport  Port=3
  EnablePWM : Inport  Port=4
  Kp_i : Inport  Port=5
  Ki_ixTcpu : Inport  Port=6
  Enable : EnablePort
  Subsystem : Subsystem
  Terminator : Terminator
  Idq_debug : Outport
  Vabc in PU : Outport  Port=2
  wires:
  Subsystem/3(VI_fb) -> Terminator/1
  Idq_ref_PU/1 -> Subsystem/3(Idq_ref_PU)
  Iab_meas_PU/1 -> Subsystem/1(Iab_meas_PU)
  EnablePWM/1 -> Subsystem/4(EnablePWM)
  Pos_PU/1 -> Subsystem/2(Pos_PU)
  Subsystem/2(VIdq_debug) -> Idq_debug/1
  Subsystem/1(Vabc in PU) -> Vabc in PU/1
  Ki_ixTcpu/1 -> Subsystem/6(Ki_ixTcpu)
  Kp_i/1 -> Subsystem/5(Kp_i)

== system Copy_of_VTOLTiltrotor/Motor Control/Controller2/Controller_MIL/F28379D Firmware/Controller Algorithm/FOC/Current Control/Control_System/Open Loop Start-Up ==
  <EnablePWM> : Inport
  SpeedRef : Inport  Port=2
  Enable : EnablePort
  3-Phase Sine Voltage Generator : mcbcontrolslib/3-Phase Sine Voltage Generator  AngleInput=Radians  N_points=1024
  Abs : Abs  SaturateOnIntegerOverflow=off
  Correction_Factor_sinePWM : Gain  Gain=2/sqrt(3)  RndMeth=Simplest  OutDataTypeStr=Inherit: Same as input
  Gain : Gain  Gain=1000
  Mux1 : Mux  Inputs=3
  PU2freq : Gain  Gain=PU_System_N_base *Maxon_645604_Np/60  RndMeth=Simplest  OutDataTypeStr=Inherit: Same as input
  Position Generator : mcbcontrolslib/Position Generator  AngleOutput=Radians  ExternalReset=none  Offset=0
  Product : Product  RndMeth=Simplest  OutDataTypeStr=Inherit: Same as first input
  Ramp Generator : Subsystem
  Ramp_Time (sec) : Constant  Value=0.0025  OutDataTypeStr=single  SampleTime=-1
  Rate Limiter : mcbcontrolslib/IIR Filter  VariantControl=Low Pass Filter  VariantSelect=Low-pass  FilterConstantInputType=Specify via dialog  Filter_constant=0.0001  advancedSettings=off  Ts=50e-6  cutOff_freq=0.31834
  Saturation : Saturate  UpperLimit=0.95  LowerLimit=0.15  RndMeth=Simplest
  V-by-f : Gain  Gain=1/(PU_System_N_base*Maxon_645604_Np*2)  RndMeth=Simplest  OutDataTypeStr=Inherit: Same as input
  position_increment : Gain  Gain=2*pi*Ts_CPU  RndMeth=Simplest  OutDataTypeStr=Inherit: Same as input
  PWM_Duty : Outport  VectorParamsAs1DForOutWhenUnconnected=off
  wires:
  3-Phase Sine Voltage Generator/1 -> Mux1/1
  3-Phase Sine Voltage Generator/3 -> Mux1/3
  Position Generator/1 -> 3-Phase Sine Voltage Generator/2  "Eps"
  Saturation/1 -> 3-Phase Sine Voltage Generator/1  "Amplitude"
  Mux1/1 -> PWM_Duty/1
  Ramp Generator/1(Ramp) -> Product/2
  Ramp_Time (sec)/1 -> Ramp Generator/1(Ramp_Time)
  Abs/1 -> V-by-f/1  "Frequency"
  position_increment/1 -> Position Generator/1
  V-by-f/1 -> Gain/1
  PU2freq/1 -> Rate Limiter/1
  Correction_Factor_sinePWM/1 -> Saturation/1
  3-Phase Sine Voltage Generator/2 -> Mux1/2
  <EnablePWM>/1 -> Ramp Generator/2(Enable)
  Product/1 -> Abs/1, position_increment/1
  Rate Limiter/1 -> Product/1
  SpeedRef/1 -> PU2freq/1
  Gain/1 -> Correction_Factor_sinePWM/1

== system Copy_of_VTOLTiltrotor/Motor Control/Controller2/Controller_MIL/F28379D Firmware/Controller Algorithm/FOC/Current Control/Control_System/Output Scaling ==
  PWM_Duty : Inport
  Enable : Inport  Port=2
  Constant : Constant  Value=0.5  OutDataTypeStr=single
  Data Type Conversion : DataTypeConversion  OutDataTypeStr=single  SaturateOnIntegerOverflow=off  RndMeth=Floor
  Gain : Gain  Gain=0.5  OutDataTypeStr=Inherit: Same as input
  Sum : Sum  Inputs=|++
  ModWave : Outport
  PWM_Enable : Outport  Port=2
  wires:
  Sum/1 -> ModWave/1  "duty"
  Constant/1 -> Sum/2
  Gain/1 -> Sum/1  "ModWave"
  PWM_Duty/1 -> Gain/1
  Data Type Conversion/1 -> PWM_Enable/1
  Enable/1 -> Data Type Conversion/1

== system Copy_of_VTOLTiltrotor/Motor Control/Controller3/Controller_MIL/F28379D Firmware/Controller Algorithm/FOC/Current Control/Control_System/Closed Loop Control ==
  Iab_meas_PU : Inport
  Pos_PU : Inport  Port=2
  Idq_ref_PU : Inport  Port=3
  EnablePWM : Inport  Port=4
  Kp_i : Inport  Port=5
  Ki_ixTcpu : Inport  Port=6
  Enable : EnablePort
  Subsystem : Subsystem
  Terminator : Terminator
  Idq_debug : Outport
  Vabc in PU : Outport  Port=2
  wires:
  Subsystem/3(VI_fb) -> Terminator/1
  Idq_ref_PU/1 -> Subsystem/3(Idq_ref_PU)
  Iab_meas_PU/1 -> Subsystem/1(Iab_meas_PU)
  EnablePWM/1 -> Subsystem/4(EnablePWM)
  Pos_PU/1 -> Subsystem/2(Pos_PU)
  Subsystem/2(VIdq_debug) -> Idq_debug/1
  Subsystem/1(Vabc in PU) -> Vabc in PU/1
  Ki_ixTcpu/1 -> Subsystem/6(Ki_ixTcpu)
  Kp_i/1 -> Subsystem/5(Kp_i)

== system Copy_of_VTOLTiltrotor/Motor Control/Controller3/Controller_MIL/F28379D Firmware/Controller Algorithm/FOC/Current Control/Control_System/Open Loop Start-Up ==
  <EnablePWM> : Inport
  SpeedRef : Inport  Port=2
  Enable : EnablePort
  3-Phase Sine Voltage Generator : mcbcontrolslib/3-Phase Sine Voltage Generator  AngleInput=Radians  N_points=1024
  Abs : Abs  SaturateOnIntegerOverflow=off
  Correction_Factor_sinePWM : Gain  Gain=2/sqrt(3)  RndMeth=Simplest  OutDataTypeStr=Inherit: Same as input
  Gain : Gain  Gain=1000
  Mux1 : Mux  Inputs=3
  PU2freq : Gain  Gain=PU_System_N_base *Maxon_645604_Np/60  RndMeth=Simplest  OutDataTypeStr=Inherit: Same as input
  Position Generator : mcbcontrolslib/Position Generator  AngleOutput=Radians  ExternalReset=none  Offset=0
  Product : Product  RndMeth=Simplest  OutDataTypeStr=Inherit: Same as first input
  Ramp Generator : Subsystem
  Ramp_Time (sec) : Constant  Value=0.0025  OutDataTypeStr=single  SampleTime=-1
  Rate Limiter : mcbcontrolslib/IIR Filter  VariantControl=Low Pass Filter  VariantSelect=Low-pass  FilterConstantInputType=Specify via dialog  Filter_constant=0.0001  advancedSettings=off  Ts=50e-6  cutOff_freq=0.31834
  Saturation : Saturate  UpperLimit=0.95  LowerLimit=0.15  RndMeth=Simplest
  V-by-f : Gain  Gain=1/(PU_System_N_base*Maxon_645604_Np*2)  RndMeth=Simplest  OutDataTypeStr=Inherit: Same as input
  position_increment : Gain  Gain=2*pi*Ts_CPU  RndMeth=Simplest  OutDataTypeStr=Inherit: Same as input
  PWM_Duty : Outport  VectorParamsAs1DForOutWhenUnconnected=off
  wires:
  3-Phase Sine Voltage Generator/1 -> Mux1/1
  3-Phase Sine Voltage Generator/3 -> Mux1/3
  Position Generator/1 -> 3-Phase Sine Voltage Generator/2  "Eps"
  Saturation/1 -> 3-Phase Sine Voltage Generator/1  "Amplitude"
  Mux1/1 -> PWM_Duty/1
  Ramp Generator/1(Ramp) -> Product/2
  Ramp_Time (sec)/1 -> Ramp Generator/1(Ramp_Time)
  Abs/1 -> V-by-f/1  "Frequency"
  position_increment/1 -> Position Generator/1
  V-by-f/1 -> Gain/1
  PU2freq/1 -> Rate Limiter/1
  Correction_Factor_sinePWM/1 -> Saturation/1
  3-Phase Sine Voltage Generator/2 -> Mux1/2
  <EnablePWM>/1 -> Ramp Generator/2(Enable)
  Product/1 -> Abs/1, position_increment/1
  Rate Limiter/1 -> Product/1
  SpeedRef/1 -> PU2freq/1
  Gain/1 -> Correction_Factor_sinePWM/1

== system Copy_of_VTOLTiltrotor/Motor Control/Controller3/Controller_MIL/F28379D Firmware/Controller Algorithm/FOC/Current Control/Control_System/Output Scaling ==
  PWM_Duty : Inport
  Enable : Inport  Port=2
  Constant : Constant  Value=0.5  OutDataTypeStr=single
  Data Type Conversion : DataTypeConversion  OutDataTypeStr=single  SaturateOnIntegerOverflow=off  RndMeth=Floor
  Gain : Gain  Gain=0.5  OutDataTypeStr=Inherit: Same as input
  Sum : Sum  Inputs=|++
  ModWave : Outport
  PWM_Enable : Outport  Port=2
  wires:
  Sum/1 -> ModWave/1  "duty"
  Constant/1 -> Sum/2
  Gain/1 -> Sum/1  "ModWave"
  PWM_Duty/1 -> Gain/1
  Data Type Conversion/1 -> PWM_Enable/1
  Enable/1 -> Data Type Conversion/1

== system Copy_of_VTOLTiltrotor/Motor Control/Controller/Controller_MIL/F28379D Firmware/Controller Algorithm/FOC/Current Control/Control_System/Closed Loop Control/Subsystem ==
  Iab_meas_PU : Inport
  Pos_PU : Inport  Port=2
  Idq_ref_PU : Inport  Port=3
  EnablePWM : Inport  Port=4
  Kp_i : Inport  Port=5
  Ki_ixTcpu : Inport  Port=6
  Clarke Transform : mcbcontrolslib/Clarke Transform  VariantControl=Variant2  PhaseInput=Two inputs  EnPowerInv=off
  Current_Controllers : Subsystem
  Demux : Demux  Outputs=2
  Inverse Park Transform : mcbcontrolslib/Inverse Park Transform  PhaseInput=Two inputs  AxisAlignment=D-axis  ThetaInput=Sine and Cosine electrical position  AngleInput=Per-unit  N_points=1024
  Mux : Mux
  Mux1 : Mux  Inputs=3
  Park Transform : mcbcontrolslib/Park Transform  PhaseInput=Two inputs  AxisAlignment=D-axis  ThetaInput=Sine and Cosine electrical position  AngleInput=Per-unit  N_points=1024
  Sine-Cosine Lookup : mcbcontrolslib/Sine-Cosine Lookup  AngleInput=Per-unit  N_points=1024  DatatypeInput=Inherit from input  Datatype=single
  Space Vector Generator : mcbcontrolslib/PWM Reference Generator  inSignal=Valphabeta  modType=SVM: space vector modulation
  Vabc in PU : Outport  VectorParamsAs1DForOutWhenUnconnected=off
  VIdq_debug : Outport  Port=2  VectorParamsAs1DForOutWhenUnconnected=off
  VI_fb : Outport  Port=3
  wires:
  Space Vector Generator/2 -> Mux1/2
  Clarke Transform/2 -> [Ibeta], Park Transform/2
  Idq_ref_PU/1 -> Current_Controllers/3(Idq_ref_PU)
  Park Transform/1 -> Current_Controllers/1(Id)
  Current_Controllers/1(Vd_ref) -> Inverse Park Transform/1
  Clarke Transform/1 -> [Ialpha], Park Transform/1
  Space Vector Generator/1 -> Mux1/1
  Iab_meas_PU/1 -> Demux/1
  Inverse Park Transform/1 -> [Valpha], Space Vector Generator/1
  Sine-Cosine Lookup/2 -> Park Transform/4, [cosTheta]
  Demux/2 -> Clarke Transform/2
  [sinTheta] -> Inverse Park Transform/3
  Park Transform/2 -> Current_Controllers/2(Iq)
  Current_Controllers/3(VIdq) -> VIdq_debug/1
  Mux1/1 -> Vabc in PU/1
  Sine-Cosine Lookup/1 -> Park Transform/3, [sinTheta]
  Demux/1 -> Clarke Transform/1
  Current_Controllers/2(Vq_ref) -> Inverse Park Transform/2
  [cosTheta] -> Inverse Park Transform/4
  Space Vector Generator/3 -> Mux1/3
  EnablePWM/1 -> Current_Controllers/4(EnablePWM)
  [Valpha] -> Mux/1
  Mux/1 -> VI_fb/1
  Pos_PU/1 -> Sine-Cosine Lookup/1
  Inverse Park Transform/2 -> [Vbeta], Space Vector Generator/2
  [Ialpha] -> Mux/3
  [Ibeta] -> Mux/4
  [Vbeta] -> Mux/2
  Ki_ixTcpu/1 -> Current_Controllers/6(Ki_ixTcpu)
  Kp_i/1 -> Current_Controllers/5(Kp_i)

== system Copy_of_VTOLTiltrotor/Motor Control/Controller/Controller_MIL/F28379D Firmware/Controller Algorithm/FOC/Current Control/Control_System/Open Loop Start-Up/Ramp Generator ==
  Ramp_Time : Inport
  Enable : Inport  Port=2
  Divide : Product  Inputs=*/  RndMeth=Simplest  OutDataTypeStr=Inherit: Same as first input
  NOT : Logic  Operator=NOT  IconShape=distinctive  AllPortsSameDT=off  OutDataTypeStr=boolean
  One : Constant  OutDataTypeStr=single  SampleTime=-1
  Ramp Generator : DiscreteIntegrator  IntegratorMethod=Accumulation: Forward Euler  gainval=1  ExternalReset=sampled level  SampleTime=-1  OutDataTypeStr=single  RndMeth=Simplest  LimitOutput=on  UpperSaturationLimit=1  LowerSaturationLimit=0  ICPrevOutput=DiscIntNeverNeededParam  ICPrevScaledInput=DiscIntNeverNeededParam
  Sample_Time : Gain  Gain=Ts_CPU  RndMeth=Simplest  OutDataTypeStr=Inherit: Same as input
  Ramp : Outport
  wires:
  Divide/1 -> Sample_Time/1
  Ramp Generator/1 -> Ramp/1  "Eps"
  Sample_Time/1 -> Ramp Generator/1
  One/1 -> Divide/1
  Ramp_Time/1 -> Divide/2
  Enable/1 -> NOT/1
  NOT/1 -> Ramp Generator/2
